simulink model "Dynamics_TranslationalEoM_TH"  (Simulink 7.8)
settings: Solver=ode45  StartTime=0.0  StopTime=10.0  RelTol=1e-3
libraries: AeroSim x1
settings Model: Creator=Ryan  LastModifiedBy=Ryan

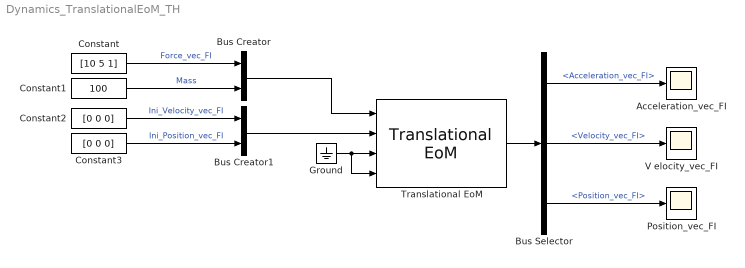
== system Dynamics_TranslationalEoM_TH ==
  Acceleration_vec_FI : Scope
  Bus Creator : BusCreator  Inputs=2
  Bus Creator1 : BusCreator  Inputs=2
  Bus Selector : BusSelector  OutputSignals=Acceleration_vec_FI,Velocity_vec_FI,Position_vec_FI
  Constant : Constant  Value=[10 5 1]
  Constant1 : Constant  Value=100
  Constant2 : Constant  Value=[0 0 0]
  Constant3 : Constant  Value=[0 0 0]
  Ground : Ground
  Position_vec_FI : Scope
      settings: SaveName=ScopeData2
  Translational EoM : AeroSim/Dynamics/Translational EoM
  V elocity_vec_FI : Scope
  wires:
  Ground/1 -> Translational EoM/4, Translational EoM/3
  Constant1/1 -> Bus Creator/2  "Mass"
  Constant/1 -> Bus Creator/1  "Force_vec_FI"
  Bus Creator/1 -> Translational EoM/1
  Constant3/1 -> Bus Creator1/2  "Ini_Position_vec_FI"
  Constant2/1 -> Bus Creator1/1  "Ini_Velocity_vec_FI"
  Bus Creator1/1 -> Translational EoM/2
  Translational EoM/1 -> Bus Selector/1
  Bus Selector/1 -> Acceleration_vec_FI/1  "<Acceleration_vec_FI>"
  Bus Selector/2 -> V elocity_vec_FI/1  "<Velocity_vec_FI>"
  Bus Selector/3 -> Position_vec_FI/1  "<Position_vec_FI>"
